simulink model "engine_control"  (Simulink 7.6)
settings: Solver=FixedStepDiscrete  StartTime=0.0  StopTime=Tfin  FixedStep=Ts  RelTol=1e-3
undefined symbols (not defined in the file or in its folder): Kd, Kp, mph2fps, throttle_trim
settings Model: Creator=borjafons  LastModifiedBy=borjafons
settings OptimizationCC: InlineParams=on  OptimizeModelRefInitCode=on  LifeSpan=1
settings DebuggingCC: FcnCallInpInsideContextMsg=Enable All
settings RTWCC: SystemTargetFile=ert.tlc  GenCodeOnly=on  TemplateMakefile=ert_default_tmf  Description=Embedded Coder  ProcessScript=ert_make_rtw_hook
settings CodeAppCC: IgnoreCustomStorageClasses=off
settings ERTTargetCC: MultiwordLength=2048  GenerateSampleERTMain=on  SupportNonFinite=off  SupportComplex=off  InlinedParameterPlacement=NonHierarchical  ERTCustomFileTemplate=example_file_process.tlc  ConvertIfToSwitch=off  SuppressUnreachableDefaultCases=off

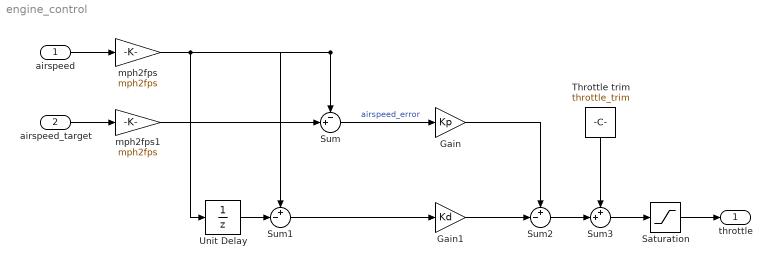
== system engine_control ==
  airspeed : Inport
  airspeed_target : Inport  Port=2
  Gain : Gain  Gain=Kp
  Gain1 : Gain  Gain=Kd
  Saturation : Saturate  UpperLimit=1  LowerLimit=.2
  Sum : Sum  Inputs=-+|
  Sum1 : Sum  Inputs=+-|
  Sum2 : Sum  Inputs=+-|
  Sum3 : Sum  Inputs=++|
  Throttle trim : Constant  Value=throttle_trim
  Unit Delay : UnitDelay  SampleTime=-1
  mph2fps : Gain  Gain=mph2fps  OutDataTypeStr=Inherit: Same as input
  mph2fps1 : Gain  Gain=mph2fps  OutDataTypeStr=Inherit: Same as input
  throttle : Outport
  wires:
  airspeed/1 -> mph2fps/1
  airspeed_target/1 -> mph2fps1/1
  Sum/1 -> Gain/1  "airspeed_error"
  Unit Delay/1 -> Sum1/2
  Sum1/1 -> Gain1/1
  Gain/1 -> Sum2/1
  Gain1/1 -> Sum2/2
  mph2fps/1 -> Unit Delay/1, Sum/1, Sum1/1
  Saturation/1 -> throttle/1
  mph2fps1/1 -> Sum/2
  Sum2/1 -> Sum3/2
  Sum3/1 -> Saturation/1
  Throttle trim/1 -> Sum3/1
